simulink model "Register_File"  (R2025b)
settings: Solver=VariableStepAuto  StartTime=0.0  StopTime=10.0  RelTol=1e-3
libraries: dspsigops x4
settings Model: Creator=cyber  LastModifiedBy=cyber

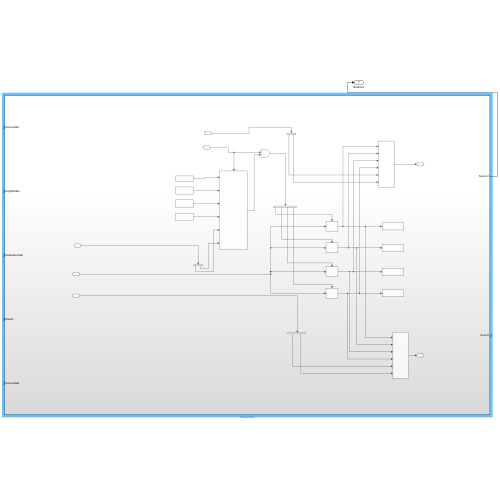
[thumbnail: Simulink's stored preview of the top-level diagram]
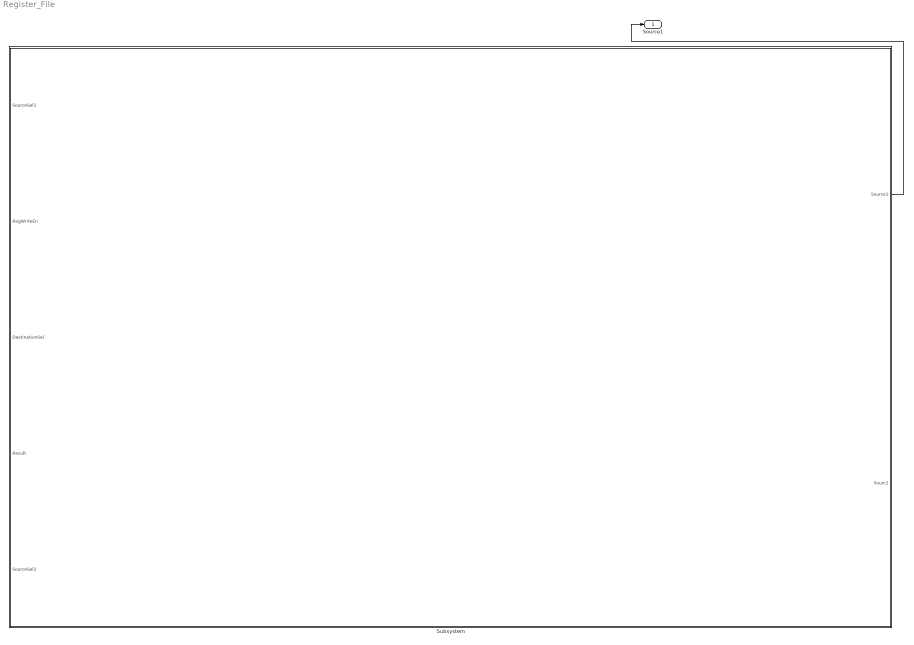
== system Register_File ==
  Subsystem : Subsystem
  Source1 : Outport
  wires:
  Subsystem/1(Source1) -> Source1/1

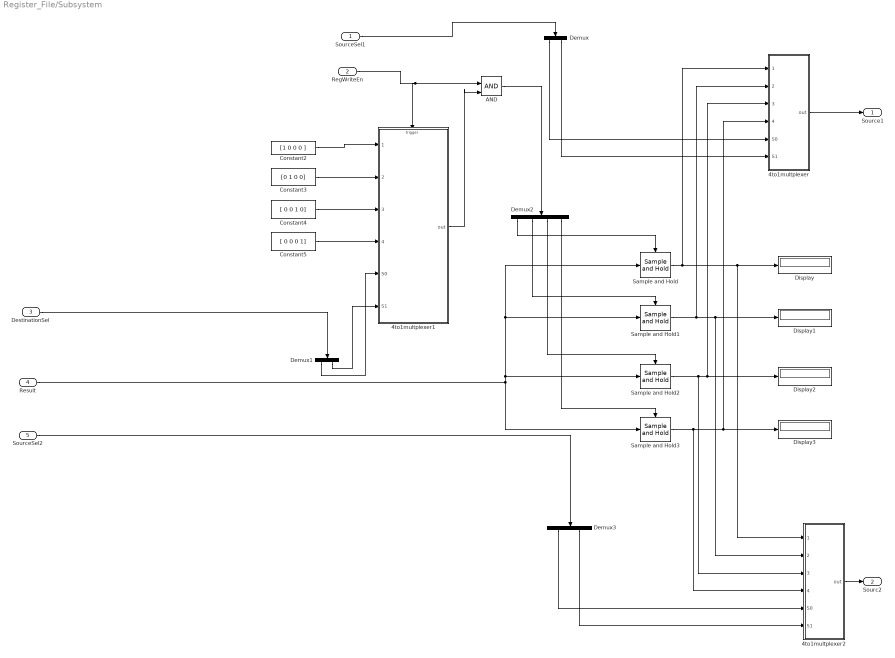
== system Register_File/Subsystem ==
  SourceSel1 : Inport
  RegWriteEn : Inport  Port=2
  DestinationSel : Inport  Port=3
  Result : Inport  Port=4
  SourceSel2 : Inport  Port=5
  4to1multplexer : Subsystem
  4to1multplexer1 : Subsystem
  4to1multplexer2 : Subsystem
  AND : Logic  IconShape=distinctive  AllPortsSameDT=off  OutDataTypeStr=boolean
  Constant2 : Constant  Value=[1 0 0 0 ]
  Constant3 : Constant  Value=[0 1 0 0]
  Constant4 : Constant  Value=[ 0 0 1 0]
  Constant5 : Constant  Value=[ 0 0 0 1]
  Demux : Demux  Outputs=2
  Demux1 : Demux  Outputs=2
  Demux2 : Demux
  Demux3 : Demux  Outputs=2
  Display{,1..3} (4 alike) : Display
  Sample and Hold{,1..3} (4 alike) : dspsigops/Sample and Hold  trig=Rising edge  initCond=0  latchinput=off
  Source1 : Outport
  Sourc2 : Outport  Port=2
  wires:
  RegWriteEn/1 -> 4to1multplexer1/Trigger, AND/1
  Demux2/4 -> Sample and Hold3/Trigger
  4to1multplexer2/1(out) -> Sourc2/1
  Sample and Hold3/1 -> 4to1multplexer2/4(4), Display3/1, 4to1multplexer/4(4)
  Sample and Hold2/1 -> 4to1multplexer2/3(3), 4to1multplexer/3(3), Display2/1
  4to1multplexer1/1(out) -> AND/2
  Result/1 -> Sample and Hold3/1, Sample and Hold/1, Sample and Hold1/1, Sample and Hold2/1
  DestinationSel/1 -> Demux1/1
  Constant4/1 -> 4to1multplexer1/3(3)
  Demux3/2 -> 4to1multplexer2/6(S1)
  Sample and Hold/1 -> 4to1multplexer/1(1), 4to1multplexer2/1(1), Display/1
  4to1multplexer/1(out) -> Source1/1
  Demux2/2 -> Sample and Hold1/Trigger
  Constant3/1 -> 4to1multplexer1/2(2)
  Demux2/3 -> Sample and Hold2/Trigger
  Demux2/1 -> Sample and Hold/Trigger
  AND/1 -> Demux2/1
  Constant5/1 -> 4to1multplexer1/4(4)
  Demux3/1 -> 4to1multplexer2/5(S0)
  Demux/2 -> 4to1multplexer/6(S1)
  SourceSel1/1 -> Demux/1
  Demux1/2 -> 4to1multplexer1/6(S1)
  Sample and Hold1/1 -> 4to1multplexer/2(2), 4to1multplexer2/2(2), Display1/1
  SourceSel2/1 -> Demux3/1
  Demux1/1 -> 4to1multplexer1/5(S0)
  Constant2/1 -> 4to1multplexer1/1(1)
  Demux/1 -> 4to1multplexer/5(S0)

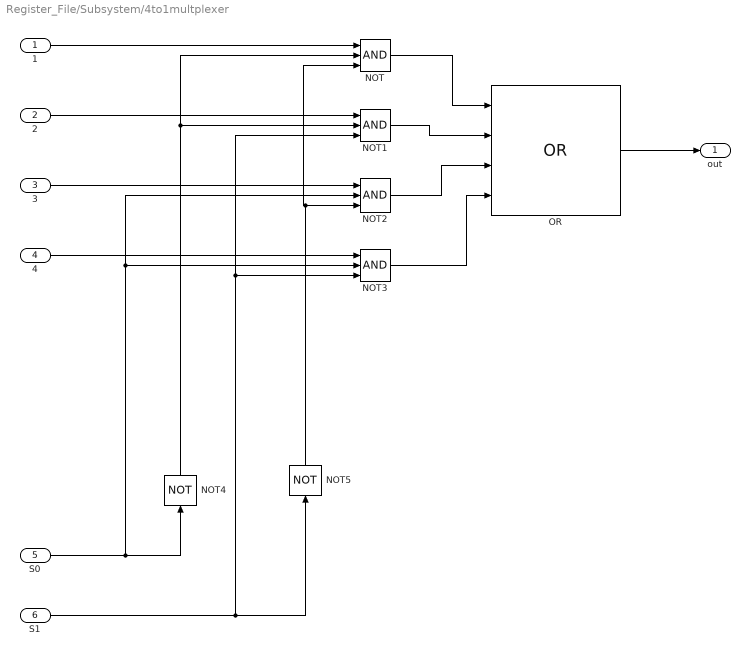
== system Register_File/Subsystem/4to1multplexer ==
  1 : Inport
  2 : Inport  Port=2
  3 : Inport  Port=3
  4 : Inport  Port=4
  S0 : Inport  Port=5
  S1 : Inport  Port=6
  NOT{,1..3} (4 alike) : Logic  Inputs=3  IconShape=distinctive  AllPortsSameDT=off  OutDataTypeStr=boolean
  NOT4 : Logic  Operator=NOT  IconShape=distinctive  AllPortsSameDT=off  OutDataTypeStr=boolean
  NOT5 : Logic  Operator=NOT  IconShape=distinctive  AllPortsSameDT=off  OutDataTypeStr=boolean
  OR : Logic  Operator=OR  Inputs=4  IconShape=distinctive  AllPortsSameDT=off  OutDataTypeStr=boolean
  out : Outport
  wires:
  NOT4/1 -> NOT/2, NOT1/2
  S1/1 -> NOT1/3, NOT3/3, NOT5/1
  NOT5/1 -> NOT/3, NOT2/3
  NOT1/1 -> OR/2
  S0/1 -> NOT4/1, NOT3/2, NOT2/2
  NOT3/1 -> OR/4
  NOT/1 -> OR/1
  NOT2/1 -> OR/3
  4/1 -> NOT3/1
  1/1 -> NOT/1
  3/1 -> NOT2/1
  2/1 -> NOT1/1
  OR/1 -> out/1

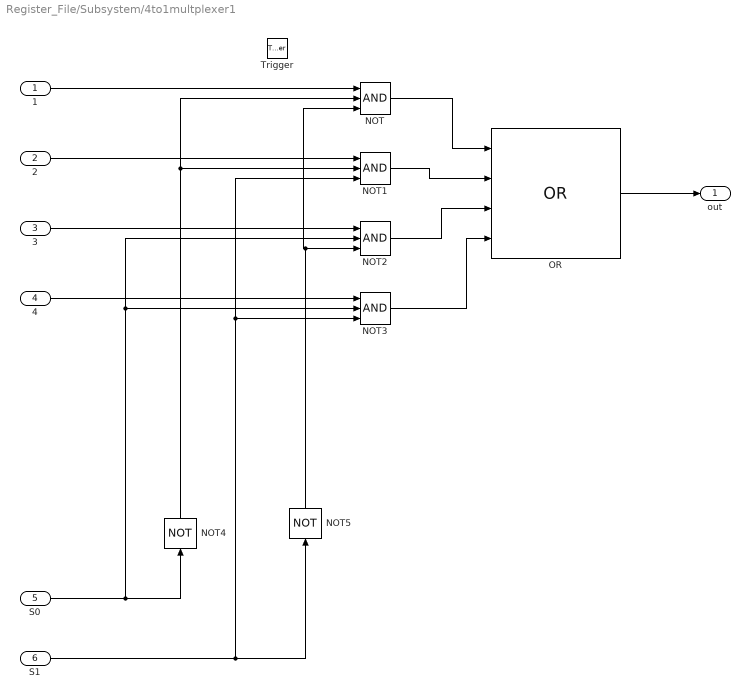
== system Register_File/Subsystem/4to1multplexer1 ==
  1 : Inport
  2 : Inport  Port=2
  3 : Inport  Port=3
  4 : Inport  Port=4
  S0 : Inport  Port=5
  S1 : Inport  Port=6
  Trigger : TriggerPort  VariantControl=(inherit)  PortDimensions=1
  NOT{,1..3} (4 alike) : Logic  Inputs=3  IconShape=distinctive  AllPortsSameDT=off  OutDataTypeStr=boolean
  NOT4 : Logic  Operator=NOT  IconShape=distinctive  AllPortsSameDT=off  OutDataTypeStr=boolean
  NOT5 : Logic  Operator=NOT  IconShape=distinctive  AllPortsSameDT=off  OutDataTypeStr=boolean
  OR : Logic  Operator=OR  Inputs=4  IconShape=distinctive  AllPortsSameDT=off  OutDataTypeStr=boolean
  out : Outport
  wires:
  NOT4/1 -> NOT/2, NOT1/2
  S1/1 -> NOT1/3, NOT3/3, NOT5/1
  NOT5/1 -> NOT/3, NOT2/3
  NOT1/1 -> OR/2
  S0/1 -> NOT4/1, NOT3/2, NOT2/2
  NOT3/1 -> OR/4
  NOT/1 -> OR/1
  NOT2/1 -> OR/3
  4/1 -> NOT3/1
  1/1 -> NOT/1
  3/1 -> NOT2/1
  2/1 -> NOT1/1
  OR/1 -> out/1

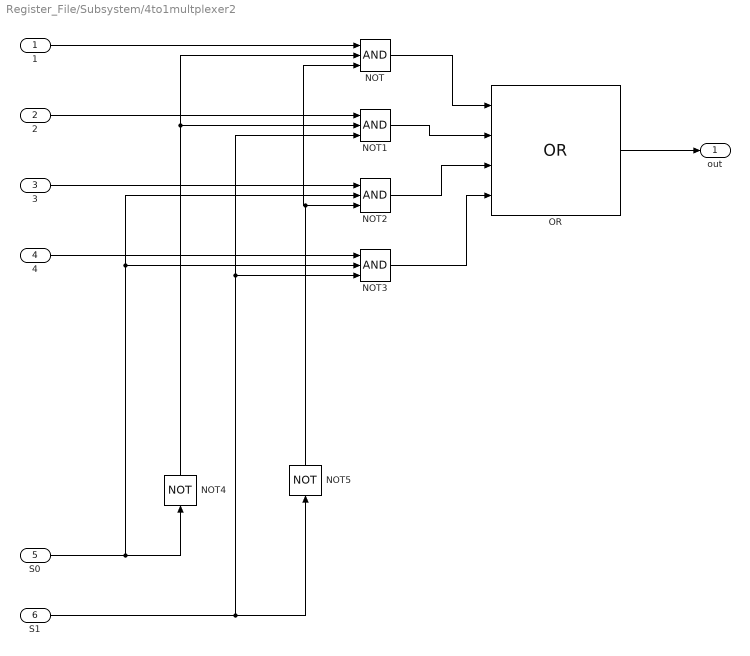
== system Register_File/Subsystem/4to1multplexer2 ==
  1 : Inport
  2 : Inport  Port=2
  3 : Inport  Port=3
  4 : Inport  Port=4
  S0 : Inport  Port=5
  S1 : Inport  Port=6
  NOT{,1..3} (4 alike) : Logic  Inputs=3  IconShape=distinctive  AllPortsSameDT=off  OutDataTypeStr=boolean
  NOT4 : Logic  Operator=NOT  IconShape=distinctive  AllPortsSameDT=off  OutDataTypeStr=boolean
  NOT5 : Logic  Operator=NOT  IconShape=distinctive  AllPortsSameDT=off  OutDataTypeStr=boolean
  OR : Logic  Operator=OR  Inputs=4  IconShape=distinctive  AllPortsSameDT=off  OutDataTypeStr=boolean
  out : Outport
  wires:
  NOT4/1 -> NOT/2, NOT1/2
  S1/1 -> NOT1/3, NOT3/3, NOT5/1
  NOT5/1 -> NOT/3, NOT2/3
  NOT1/1 -> OR/2
  S0/1 -> NOT4/1, NOT3/2, NOT2/2
  NOT3/1 -> OR/4
  NOT/1 -> OR/1
  NOT2/1 -> OR/3
  4/1 -> NOT3/1
  1/1 -> NOT/1
  3/1 -> NOT2/1
  2/1 -> NOT1/1
  OR/1 -> out/1
